simulink model "data_generator_plant"  (R2013a)
settings: Solver=ode45  StartTime=0.0  StopTime=1000  RelTol=1e-3
libraries: cstblocks x3, simulink x1
settings Model: Creator=melanholly  LastModifiedBy=melanholly

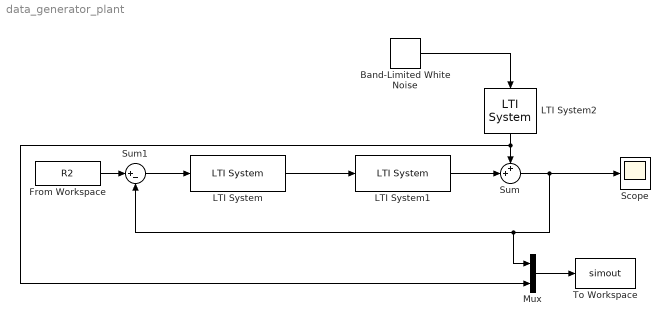
== system data_generator_plant ==
  Band-Limited White Noise : simulink/Sources/Band-Limited White Noise  Cov=[0.00001]  Ts=0.1  seed=[054651321650]
  From Workspace : FromWorkspace  VariableName=R2  SampleTime=0
  LTI System : cstblocks/LTI System  sys=C  IC=[]
  LTI System1 : cstblocks/LTI System  sys=G0  IC=[]
  LTI System2 : cstblocks/LTI System  sys=H0  IC=[]
  Mux : Mux  Inputs=2
  Scope : Scope
  Sum : Sum  Inputs=++|
  Sum1 : Sum  Inputs=|+-
  To Workspace : ToWorkspace  VariableName=simout  SampleTime=-1
  wires:
  LTI System2/1 -> Mux/2, Sum/1
  LTI System1/1 -> Sum/2
  LTI System/1 -> LTI System1/1
  Sum1/1 -> LTI System/1
  From Workspace/1 -> Sum1/1
  Sum/1 -> Mux/1, Sum1/2, Scope/1
  Band-Limited White Noise/1 -> LTI System2/1
  Mux/1 -> To Workspace/1
